simulink model "IEEE30_case"  (R2024b)
settings: Solver=FixedStepAuto  StartTime=0  StopTime=5  FixedStep=1e-7  RelTol=1e-3
values from neighbouring files (symbols this model uses):
  GFL_DFIG_7_C_bus = 0.08    [IEEE30_case_parameters.m]
  GFL_DFIG_7_D_mutual = 2.500000e+3    (= 2500)    [IEEE30_case_parameters.m]
  GFL_DFIG_7_f0 = 60    [IEEE30_case_parameters.m]
  GFL_DFIG_7_gPLLi = 3200    [IEEE30_case_parameters.m]
  GFL_DFIG_7_gPLLp = 650    [IEEE30_case_parameters.m]
  GFL_DFIG_7_H_WT = 0.4    [IEEE30_case_parameters.m]
  GFL_DFIG_7_Hg = 0.8    [IEEE30_case_parameters.m]
  GFL_DFIG_7_Igq_ref = 0    [IEEE30_case_parameters.m]
  GFL_DFIG_7_Ird_ref = 704.45696    [IEEE30_case_parameters.m]
  GFL_DFIG_7_KI_V = -300000    [IEEE30_case_parameters.m]
  GFL_DFIG_7_KP_V = -1000    [IEEE30_case_parameters.m]
  GFL_DFIG_7_Ksh = 1.254300e+4    (= 12543)    [IEEE30_case_parameters.m]
  GFL_DFIG_7_Lg = 0.000483    [IEEE30_case_parameters.m]
  GFL_DFIG_7_Lm_pu = 4    [IEEE30_case_parameters.m]
  GFL_DFIG_7_N = 100    [IEEE30_case_parameters.m]
  GFL_DFIG_7_p = 2    [IEEE30_case_parameters.m]
  GFL_DFIG_7_Pitch = 0    [IEEE30_case_parameters.m]
  GFL_DFIG_7_R = 44    [IEEE30_case_parameters.m]
  GFL_DFIG_7_Rg = 2.000000e-5    (= 2e-05)    [IEEE30_case_parameters.m]
  GFL_DFIG_7_rho = 1.225    [IEEE30_case_parameters.m]
  GFL_DFIG_7_rPLLi = 4500    [IEEE30_case_parameters.m]
  GFL_DFIG_7_rPLLp = 620    [IEEE30_case_parameters.m]
  GFL_DFIG_7_Rs_pu = 0.011    [IEEE30_case_parameters.m]
  GFL_DFIG_7_Sbase = 2.000000e+6    (= 2000000)    [IEEE30_case_parameters.m]
  GFL_DFIG_7_ugq_ref = 0    [IEEE30_case_parameters.m]
  GFL_DFIG_7_usd_ref = 0    [IEEE30_case_parameters.m]
  GFL_DFIG_7_Vbase = 690    [IEEE30_case_parameters.m]
  GFL_DFIG_7_Vdc_ref = 1200    [IEEE30_case_parameters.m]
  GFL_DFIG_7_wind = 12    [IEEE30_case_parameters.m]
  GFL_DFIG_7_wm_ref = 518.184209    [IEEE30_case_parameters.m]
  SG_D_13_D = 0.01056    [IEEE30_case_parameters.m]
  SG_D_13_EnableSaturation = 0    [IEEE30_case_parameters.m]
  SG_D_13_f0 = 60    [IEEE30_case_parameters.m]
  SG_D_13_H = 7.5    [IEEE30_case_parameters.m]
  SG_D_13_K_A = 20    [IEEE30_case_parameters.m]
  SG_D_13_K_E = 1.000000e+1    (= 10)    [IEEE30_case_parameters.m]
  SG_D_13_K_F = 2.363    [IEEE30_case_parameters.m]
  SG_D_13_K_s = 0.5    [IEEE30_case_parameters.m]
  SG_D_13_R_a = 0.001088    [IEEE30_case_parameters.m]
  SG_D_13_S_A = 1    [IEEE30_case_parameters.m]
  SG_D_13_S_B = 0.103    [IEEE30_case_parameters.m]
  SG_D_13_S_N = 10.659857    [IEEE30_case_parameters.m]
  SG_D_13_SpeedPara = 200    [IEEE30_case_parameters.m]
  SG_D_13_T_0 = 0.370163    [IEEE30_case_parameters.m]
  SG_D_13_T_1 = 0.3    [IEEE30_case_parameters.m]
  SG_D_13_T_2 = 0.05    [IEEE30_case_parameters.m]
  SG_D_13_T_3 = 0.02    [IEEE30_case_parameters.m]
  SG_D_13_T_4 = 0.005    [IEEE30_case_parameters.m]
  SG_D_13_T_A = 0.02    [IEEE30_case_parameters.m]
  SG_D_13_T_dd = 8.000000e+0    (= 8)    [IEEE30_case_parameters.m]
  SG_D_13_T_ddd = 0.04    [IEEE30_case_parameters.m]
  SG_D_13_T_E = 0.314    [IEEE30_case_parameters.m]
  SG_D_13_T_F = 0.35    [IEEE30_case_parameters.m]
  SG_D_13_T_qd = 0.8    [IEEE30_case_parameters.m]
  SG_D_13_T_qdd = 0.02    [IEEE30_case_parameters.m]
  SG_D_13_T_speed = 0.1    [IEEE30_case_parameters.m]
  SG_D_13_T_w = 0.5    [IEEE30_case_parameters.m]
  SG_D_13_V_ref = 1.696619    [IEEE30_case_parameters.m]
  SG_D_13_w_ref = 376.991118    [IEEE30_case_parameters.m]
  SG_D_13_x_d = 1.9    [IEEE30_case_parameters.m]
  SG_D_13_x_dd = 0.302    [IEEE30_case_parameters.m]
  SG_D_13_x_ddd = 0.204    [IEEE30_case_parameters.m]
  SG_D_13_x_l = 0.05    [IEEE30_case_parameters.m]
  SG_D_13_x_q = 1.3    [IEEE30_case_parameters.m]
  SG_D_13_x_qd = 0.5    [IEEE30_case_parameters.m]
  SG_D_13_x_qdd = 0.3    [IEEE30_case_parameters.m]
  SG_D_1_D = 0.01056    [IEEE30_case_parameters.m]
  SG_D_1_EnableSaturation = 0    [IEEE30_case_parameters.m]
  SG_D_1_f0 = 60    [IEEE30_case_parameters.m]
  SG_D_1_H = 7.5    [IEEE30_case_parameters.m]
  SG_D_1_K_A = 20    [IEEE30_case_parameters.m]
  SG_D_1_K_E = 1.000000e+1    (= 10)    [IEEE30_case_parameters.m]
  SG_D_1_K_F = 2.363    [IEEE30_case_parameters.m]
  SG_D_1_K_s = 0.5    [IEEE30_case_parameters.m]
  SG_D_1_R_a = 0.001088    [IEEE30_case_parameters.m]
  SG_D_1_S_A = 1    [IEEE30_case_parameters.m]
  SG_D_1_S_B = 0.103    [IEEE30_case_parameters.m]
  SG_D_1_S_N = 10.659857    [IEEE30_case_parameters.m]
  SG_D_1_SpeedPara = 200    [IEEE30_case_parameters.m]
  SG_D_1_T_0 = 0.259812    [IEEE30_case_parameters.m]
  SG_D_1_T_1 = 0.3    [IEEE30_case_parameters.m]
  SG_D_1_T_2 = 0.05    [IEEE30_case_parameters.m]
  SG_D_1_T_3 = 0.02    [IEEE30_case_parameters.m]
  SG_D_1_T_4 = 0.005    [IEEE30_case_parameters.m]
  SG_D_1_T_A = 0.02    [IEEE30_case_parameters.m]
  SG_D_1_T_dd = 8.000000e+0    (= 8)    [IEEE30_case_parameters.m]
  SG_D_1_T_ddd = 0.04    [IEEE30_case_parameters.m]
  SG_D_1_T_E = 0.314    [IEEE30_case_parameters.m]
  SG_D_1_T_F = 0.35    [IEEE30_case_parameters.m]
  SG_D_1_T_qd = 0.8    [IEEE30_case_parameters.m]
  SG_D_1_T_qdd = 0.02    [IEEE30_case_parameters.m]
  SG_D_1_T_speed = 0.1    [IEEE30_case_parameters.m]
  SG_D_1_T_w = 0.5    [IEEE30_case_parameters.m]
  SG_D_1_V_ref = 1.544107    [IEEE30_case_parameters.m]
  SG_D_1_w_ref = 376.991118    [IEEE30_case_parameters.m]
  SG_D_1_x_d = 1.9    [IEEE30_case_parameters.m]
  SG_D_1_x_dd = 0.302    [IEEE30_case_parameters.m]
  SG_D_1_x_ddd = 0.204    [IEEE30_case_parameters.m]
  SG_D_1_x_l = 0.05    [IEEE30_case_parameters.m]
  SG_D_1_x_q = 1.3    [IEEE30_case_parameters.m]
  SG_D_1_x_qd = 0.5    [IEEE30_case_parameters.m]
  SG_D_1_x_qdd = 0.3    [IEEE30_case_parameters.m]
  SG_D_22_D = 0.01056    [IEEE30_case_parameters.m]
  SG_D_22_EnableSaturation = 0    [IEEE30_case_parameters.m]
  SG_D_22_f0 = 60    [IEEE30_case_parameters.m]
  SG_D_22_H = 7.5    [IEEE30_case_parameters.m]
  SG_D_22_K_A = 20    [IEEE30_case_parameters.m]
  SG_D_22_K_E = 1.000000e+1    (= 10)    [IEEE30_case_parameters.m]
  SG_D_22_K_F = 2.363    [IEEE30_case_parameters.m]
  SG_D_22_K_s = 0.5    [IEEE30_case_parameters.m]
  SG_D_22_R_a = 0.001088    [IEEE30_case_parameters.m]
  SG_D_22_S_A = 1    [IEEE30_case_parameters.m]
  SG_D_22_S_B = 0.103    [IEEE30_case_parameters.m]
  SG_D_22_S_N = 10.659857    [IEEE30_case_parameters.m]
  SG_D_22_SpeedPara = 200    [IEEE30_case_parameters.m]
  SG_D_22_T_0 = 0.216121    [IEEE30_case_parameters.m]
  SG_D_22_T_1 = 0.3    [IEEE30_case_parameters.m]
  SG_D_22_T_2 = 0.05    [IEEE30_case_parameters.m]
  SG_D_22_T_3 = 0.02    [IEEE30_case_parameters.m]
  SG_D_22_T_4 = 0.005    [IEEE30_case_parameters.m]
  ... (+126 more)
(part 4 of 27)

== system IEEE30_case/SG_D_22 ==
  v_d_SG_D_22 : Inport
  v_q_SG_D_22 : Inport  Port=2
  E_fd_SG_D_22 : Integrator  InitialCondition=1.7973763049191707
  Px_1_SG_D_22 : Integrator  InitialCondition=0.0
  Px_2_SG_D_22 : Integrator  InitialCondition=0.0
  Px_3_SG_D_22 : Integrator  InitialCondition=9.720418694266681e-32
  R_f_SG_D_22 : Integrator  InitialCondition=12.134857738640001
  T_e_SG_D_22_block : Subsystem
  T_m_SG_D_22 : Integrator  InitialCondition=0.21612107186011983
  V_f_SG_D_22 : Integrator  InitialCondition=17.973763049191707
  d_E_fd_SG_D_22_block : Subsystem
  d_Px_1_SG_D_22_block : Subsystem
  d_Px_2_SG_D_22_block : Subsystem
  d_Px_3_SG_D_22_block : Subsystem
  d_R_f_SG_D_22_block : Subsystem
  d_T_m_SG_D_22_block : Subsystem
  d_V_f_SG_D_22_block : Subsystem
  d_psi_1d_SG_D_22_block : Subsystem
  d_psi_d_SG_D_22_block : Subsystem
  d_psi_fd_SG_D_22_block : Subsystem
  d_psi_gq_SG_D_22_block : Subsystem
  d_psi_kq_SG_D_22_block : Subsystem
  d_psi_q_SG_D_22_block : Subsystem
  d_theta_SG_D_22_block : Subsystem
  d_w_SG_D_22_block : Subsystem
  i_d_SG_D_22_block : Subsystem
  i_q_SG_D_22_block : Subsystem
  psi_1d_SG_D_22 : Integrator  InitialCondition=1.00488248469618
  psi_d_SG_D_22 : Integrator  InitialCondition=0.9834637327982612
  psi_fd_SG_D_22 : Integrator  InitialCondition=1.11283299426169
  psi_gq_SG_D_22 : Integrator  InitialCondition=0.11224508298484515
  psi_kq_SG_D_22 : Integrator  InitialCondition=-0.17538294216382055
  psi_q_SG_D_22 : Integrator  InitialCondition=-0.18239825985037336
  theta_SG_D_22 : Integrator  InitialCondition=0.1237367846423987
  theta_SG_D_22_out_block : Subsystem
  w_SG_D_22 : Integrator  InitialCondition=376.99111843077515
  w_SG_D_22_out_block : Subsystem
  i_d_SG_D_22 : Outport
  i_q_SG_D_22 : Outport  Port=2
  T_e_SG_D_22 : Outport  Port=3
  w_SG_D_22_out : Outport  Port=4
  theta_SG_D_22_out : Outport  Port=5
  wires:
  d_T_m_SG_D_22_block/1(Blockout_d_T_m_SG_D_22_e6732) -> T_m_SG_D_22/1
  psi_kq_SG_D_22/1 -> d_psi_gq_SG_D_22_block/3(State_psi_kq_SG_D_22_f3021), d_psi_q_SG_D_22_block/2(State_psi_kq_SG_D_22_098fe), d_psi_gq_SG_D_22_block/5(State_psi_kq_SG_D_22_d52e6), d_psi_gq_SG_D_22_block/8(State_psi_kq_SG_D_22_c01c1), d_psi_kq_SG_D_22_block/2(State_psi_kq_SG_D_22_eb2c5), i_d_SG_D_22_block/2(State_psi_kq_SG_D_22_d07e7), d_V_f_SG_D_22_block/10(State_psi_kq_SG_D_22_352c2), i_q_SG_D_22_block/2(State_psi_kq_SG_D_22_c8bb0), d_w_SG_D_22_block/5(State_psi_kq_SG_D_22_23ee7), d_psi_kq_SG_D_22_block/4(State_psi_kq_SG_D_22_49ea5), T_e_SG_D_22_block/3(State_psi_kq_SG_D_22_80cd8)
  w_SG_D_22/1 -> d_psi_d_SG_D_22_block/9(State_w_SG_D_22_ad5b4), d_psi_q_SG_D_22_block/9(State_w_SG_D_22_27ecd), d_w_SG_D_22_block/1(State_w_SG_D_22_fa999), d_V_f_SG_D_22_block/13(State_w_SG_D_22_31356), d_V_f_SG_D_22_block/8(State_w_SG_D_22_d59fe), d_theta_SG_D_22_block/1(State_w_SG_D_22_7f5ca), d_T_m_SG_D_22_block/1(State_w_SG_D_22_92dc5), d_Px_1_SG_D_22_block/2(State_w_SG_D_22_b06b5), d_Px_2_SG_D_22_block/4(State_w_SG_D_22_79a8a), d_Px_3_SG_D_22_block/6(State_w_SG_D_22_b3bb6), w_SG_D_22_out_block/1(State_w_SG_D_22_6ca8a)
  d_Px_1_SG_D_22_block/1(Blockout_d_Px_1_SG_D_22_5a954) -> Px_1_SG_D_22/1
  i_q_SG_D_22_block/1(Blockout_i_q_SG_D_22_b8c62) -> i_q_SG_D_22/1
  T_e_SG_D_22_block/1(Blockout_T_e_SG_D_22_9d77c) -> T_e_SG_D_22/1
  psi_gq_SG_D_22/1 -> d_psi_q_SG_D_22_block/1(State_psi_gq_SG_D_22_8eb30), d_psi_gq_SG_D_22_block/1(State_psi_gq_SG_D_22_18129), d_psi_gq_SG_D_22_block/2(State_psi_gq_SG_D_22_c69e2), d_psi_gq_SG_D_22_block/4(State_psi_gq_SG_D_22_61da9), d_psi_kq_SG_D_22_block/1(State_psi_gq_SG_D_22_5f63f), i_d_SG_D_22_block/1(State_psi_gq_SG_D_22_058cc), d_V_f_SG_D_22_block/9(State_psi_gq_SG_D_22_abe45), d_w_SG_D_22_block/4(State_psi_gq_SG_D_22_bb4d3), i_q_SG_D_22_block/1(State_psi_gq_SG_D_22_6529e), d_psi_kq_SG_D_22_block/3(State_psi_gq_SG_D_22_c1d1e), d_psi_gq_SG_D_22_block/7(State_psi_gq_SG_D_22_1b6c4), T_e_SG_D_22_block/2(State_psi_gq_SG_D_22_ecb3d)
  v_q_SG_D_22/1 -> d_psi_d_SG_D_22_block/6(Input_v_q_SG_D_22_3bdb8), d_psi_q_SG_D_22_block/6(Input_v_q_SG_D_22_03d27)
  d_theta_SG_D_22_block/1(Blockout_d_theta_SG_D_22_65d2b) -> theta_SG_D_22/1
  d_Px_3_SG_D_22_block/1(Blockout_d_Px_3_SG_D_22_a3854) -> Px_3_SG_D_22/1
  theta_SG_D_22_out_block/1(Blockout_theta_SG_D_22_out_cf0c5) -> theta_SG_D_22_out/1
  d_Px_2_SG_D_22_block/1(Blockout_d_Px_2_SG_D_22_87151) -> Px_2_SG_D_22/1
  w_SG_D_22_out_block/1(Blockout_w_SG_D_22_out_8ba47) -> w_SG_D_22_out/1
  psi_1d_SG_D_22/1 -> d_psi_fd_SG_D_22_block/3(State_psi_1d_SG_D_22_be8ba), d_psi_fd_SG_D_22_block/8(State_psi_1d_SG_D_22_ea7d2), d_psi_d_SG_D_22_block/1(State_psi_1d_SG_D_22_f0d35), d_psi_1d_SG_D_22_block/1(State_psi_1d_SG_D_22_172da), d_V_f_SG_D_22_block/4(State_psi_1d_SG_D_22_11dba), d_psi_1d_SG_D_22_block/3(State_psi_1d_SG_D_22_e0ab6), d_w_SG_D_22_block/8(State_psi_1d_SG_D_22_62d4d), i_d_SG_D_22_block/5(State_psi_1d_SG_D_22_424d2), d_psi_fd_SG_D_22_block/5(State_psi_1d_SG_D_22_63a8d), i_q_SG_D_22_block/5(State_psi_1d_SG_D_22_666cb), T_e_SG_D_22_block/6(State_psi_1d_SG_D_22_9ed94)
  Px_3_SG_D_22/1 -> d_V_f_SG_D_22_block/3(State_Px_3_SG_D_22_7a9b4), d_Px_3_SG_D_22_block/1(State_Px_3_SG_D_22_2d550)
  theta_SG_D_22/1 -> d_psi_d_SG_D_22_block/5(State_theta_SG_D_22_96219), d_psi_d_SG_D_22_block/7(State_theta_SG_D_22_18f7d), d_psi_q_SG_D_22_block/5(State_theta_SG_D_22_55bda), i_d_SG_D_22_block/4(State_theta_SG_D_22_792f8), i_d_SG_D_22_block/8(State_theta_SG_D_22_e389e), i_q_SG_D_22_block/4(State_theta_SG_D_22_35a4e), i_q_SG_D_22_block/8(State_theta_SG_D_22_5c4fb), theta_SG_D_22_out_block/1(State_theta_SG_D_22_89d34), d_psi_q_SG_D_22_block/7(State_theta_SG_D_22_3fd59)
  Px_2_SG_D_22/1 -> d_Px_3_SG_D_22_block/2(State_Px_2_SG_D_22_afba3), d_Px_3_SG_D_22_block/3(State_Px_2_SG_D_22_1a197), d_Px_2_SG_D_22_block/1(State_Px_2_SG_D_22_a7e01)
  d_psi_kq_SG_D_22_block/1(Blockout_d_psi_kq_SG_D_22_a4b99) -> psi_kq_SG_D_22/1
  psi_d_SG_D_22/1 -> d_psi_fd_SG_D_22_block/9(State_psi_d_SG_D_22_f7c75), d_psi_fd_SG_D_22_block/6(State_psi_d_SG_D_22_1ab68), d_psi_d_SG_D_22_block/2(State_psi_d_SG_D_22_c5170), d_psi_q_SG_D_22_block/8(State_psi_d_SG_D_22_a1733), d_psi_1d_SG_D_22_block/4(State_psi_d_SG_D_22_a4972), d_w_SG_D_22_block/3(State_psi_d_SG_D_22_73560), d_V_f_SG_D_22_block/5(State_psi_d_SG_D_22_b21fa), d_w_SG_D_22_block/9(State_psi_d_SG_D_22_0b647), i_q_SG_D_22_block/6(State_psi_d_SG_D_22_f015b), i_d_SG_D_22_block/6(State_psi_d_SG_D_22_8fd04), T_e_SG_D_22_block/1(State_psi_d_SG_D_22_b0899), T_e_SG_D_22_block/7(State_psi_d_SG_D_22_2f3ed), d_V_f_SG_D_22_block/12(State_psi_d_SG_D_22_8b3f8)
  T_m_SG_D_22/1 -> d_T_m_SG_D_22_block/2(State_T_m_SG_D_22_f2698), d_w_SG_D_22_block/2(State_T_m_SG_D_22_7e244)
  v_d_SG_D_22/1 -> d_psi_d_SG_D_22_block/4(Input_v_d_SG_D_22_73bdd), d_psi_q_SG_D_22_block/4(Input_v_d_SG_D_22_2b34c)
  i_d_SG_D_22_block/1(Blockout_i_d_SG_D_22_9977f) -> i_d_SG_D_22/1
  psi_fd_SG_D_22/1 -> d_psi_fd_SG_D_22_block/4(State_psi_fd_SG_D_22_f44ac), d_psi_fd_SG_D_22_block/7(State_psi_fd_SG_D_22_b3331), d_psi_fd_SG_D_22_block/10(State_psi_fd_SG_D_22_ee685), d_psi_fd_SG_D_22_block/2(State_psi_fd_SG_D_22_5b8ee), d_psi_d_SG_D_22_block/3(State_psi_fd_SG_D_22_05db2), d_psi_1d_SG_D_22_block/2(State_psi_fd_SG_D_22_c2d5a), d_V_f_SG_D_22_block/6(State_psi_fd_SG_D_22_e3f07), i_d_SG_D_22_block/7(State_psi_fd_SG_D_22_0bdd4), d_w_SG_D_22_block/10(State_psi_fd_SG_D_22_b8daa), d_psi_1d_SG_D_22_block/5(State_psi_fd_SG_D_22_3322a), i_q_SG_D_22_block/7(State_psi_fd_SG_D_22_6d852), T_e_SG_D_22_block/8(State_psi_fd_SG_D_22_d61c9)
  psi_q_SG_D_22/1 -> d_psi_d_SG_D_22_block/8(State_psi_q_SG_D_22_e1063), d_psi_q_SG_D_22_block/3(State_psi_q_SG_D_22_dc44e), d_psi_gq_SG_D_22_block/6(State_psi_q_SG_D_22_52758), d_psi_gq_SG_D_22_block/9(State_psi_q_SG_D_22_91585), d_psi_kq_SG_D_22_block/5(State_psi_q_SG_D_22_89f21), d_w_SG_D_22_block/6(State_psi_q_SG_D_22_4ef4a), d_V_f_SG_D_22_block/7(State_psi_q_SG_D_22_f5df1), d_V_f_SG_D_22_block/11(State_psi_q_SG_D_22_c4168), d_w_SG_D_22_block/7(State_psi_q_SG_D_22_8c90d), i_d_SG_D_22_block/3(State_psi_q_SG_D_22_9e84b), T_e_SG_D_22_block/5(State_psi_q_SG_D_22_21d92), T_e_SG_D_22_block/4(State_psi_q_SG_D_22_f98a6), i_q_SG_D_22_block/3(State_psi_q_SG_D_22_a1550)
  Px_1_SG_D_22/1 -> d_Px_2_SG_D_22_block/2(State_Px_1_SG_D_22_e638c), d_Px_3_SG_D_22_block/4(State_Px_1_SG_D_22_68613), d_Px_3_SG_D_22_block/5(State_Px_1_SG_D_22_83b83), d_Px_2_SG_D_22_block/3(State_Px_1_SG_D_22_dd336), d_Px_1_SG_D_22_block/1(State_Px_1_SG_D_22_97642)
  d_E_fd_SG_D_22_block/1(Blockout_d_E_fd_SG_D_22_040cd) -> E_fd_SG_D_22/1
  d_V_f_SG_D_22_block/1(Blockout_d_V_f_SG_D_22_187ed) -> V_f_SG_D_22/1
  d_psi_1d_SG_D_22_block/1(Blockout_d_psi_1d_SG_D_22_39dbc) -> psi_1d_SG_D_22/1
  d_R_f_SG_D_22_block/1(Blockout_d_R_f_SG_D_22_62abf) -> R_f_SG_D_22/1
  d_psi_gq_SG_D_22_block/1(Blockout_d_psi_gq_SG_D_22_8bac2) -> psi_gq_SG_D_22/1
  d_psi_d_SG_D_22_block/1(Blockout_d_psi_d_SG_D_22_244d3) -> psi_d_SG_D_22/1
  d_w_SG_D_22_block/1(Blockout_d_w_SG_D_22_fc61f) -> w_SG_D_22/1
  d_psi_q_SG_D_22_block/1(Blockout_d_psi_q_SG_D_22_d620a) -> psi_q_SG_D_22/1
  R_f_SG_D_22/1 -> d_V_f_SG_D_22_block/2(State_R_f_SG_D_22_2faca), d_R_f_SG_D_22_block/2(State_R_f_SG_D_22_53fbc)
  V_f_SG_D_22/1 -> d_V_f_SG_D_22_block/14(State_V_f_SG_D_22_db965), d_E_fd_SG_D_22_block/2(State_V_f_SG_D_22_c66fa)
  E_fd_SG_D_22/1 -> d_V_f_SG_D_22_block/1(State_E_fd_SG_D_22_743c3), d_E_fd_SG_D_22_block/1(State_E_fd_SG_D_22_b7fa0), d_psi_fd_SG_D_22_block/1(State_E_fd_SG_D_22_516e7), d_R_f_SG_D_22_block/1(State_E_fd_SG_D_22_1081a)
  d_psi_fd_SG_D_22_block/1(Blockout_d_psi_fd_SG_D_22_1ac55) -> psi_fd_SG_D_22/1

== system IEEE30_case/SG_D_23 ==
  v_d_SG_D_23 : Inport
  v_q_SG_D_23 : Inport  Port=2
  E_fd_SG_D_23 : Integrator  InitialCondition=1.2033630369488155
  Px_1_SG_D_23 : Integrator  InitialCondition=0.0
  Px_2_SG_D_23 : Integrator  InitialCondition=0.0
  Px_3_SG_D_23 : Integrator  InitialCondition=-1.0345427304101987e-30
  R_f_SG_D_23 : Integrator  InitialCondition=8.124419589457288
  T_e_SG_D_23_block : Subsystem
  T_m_SG_D_23 : Integrator  InitialCondition=0.19204698605794301
  V_f_SG_D_23 : Integrator  InitialCondition=12.033630369488154
  d_E_fd_SG_D_23_block : Subsystem
  d_Px_1_SG_D_23_block : Subsystem
  d_Px_2_SG_D_23_block : Subsystem
  d_Px_3_SG_D_23_block : Subsystem
  d_R_f_SG_D_23_block : Subsystem
  d_T_m_SG_D_23_block : Subsystem
  d_V_f_SG_D_23_block : Subsystem
  d_psi_1d_SG_D_23_block : Subsystem
  d_psi_d_SG_D_23_block : Subsystem
  d_psi_fd_SG_D_23_block : Subsystem
  d_psi_gq_SG_D_23_block : Subsystem
  d_psi_kq_SG_D_23_block : Subsystem
  d_psi_q_SG_D_23_block : Subsystem
  d_theta_SG_D_23_block : Subsystem
  d_w_SG_D_23_block : Subsystem
  i_d_SG_D_23_block : Subsystem
  i_q_SG_D_23_block : Subsystem
  psi_1d_SG_D_23 : Integrator  InitialCondition=0.9815595669546187
  psi_d_SG_D_23 : Integrator  InitialCondition=0.975564878576397
  psi_fd_SG_D_23 : Integrator  InitialCondition=1.0117727963808552
  psi_gq_SG_D_23 : Integrator  InitialCondition=0.13579101365568608
  psi_kq_SG_D_23 : Integrator  InitialCondition=-0.2121734588370095
  psi_q_SG_D_23 : Integrator  InitialCondition=-0.22066039719048988
  theta_SG_D_23 : Integrator  InitialCondition=0.19462050662964567
  theta_SG_D_23_out_block : Subsystem
  w_SG_D_23 : Integrator  InitialCondition=376.99111843077515
  w_SG_D_23_out_block : Subsystem
  i_d_SG_D_23 : Outport
  i_q_SG_D_23 : Outport  Port=2
  T_e_SG_D_23 : Outport  Port=3
  w_SG_D_23_out : Outport  Port=4
  theta_SG_D_23_out : Outport  Port=5
  wires:
  theta_SG_D_23/1 -> d_psi_d_SG_D_23_block/5(State_theta_SG_D_23_2ec18), d_psi_q_SG_D_23_block/7(State_theta_SG_D_23_99733), i_d_SG_D_23_block/4(State_theta_SG_D_23_46601), i_q_SG_D_23_block/4(State_theta_SG_D_23_c31a3), d_psi_q_SG_D_23_block/5(State_theta_SG_D_23_d0e02), d_psi_d_SG_D_23_block/7(State_theta_SG_D_23_794b5), theta_SG_D_23_out_block/1(State_theta_SG_D_23_9d978), i_q_SG_D_23_block/8(State_theta_SG_D_23_c16ba), i_d_SG_D_23_block/8(State_theta_SG_D_23_15384)
  w_SG_D_23/1 -> d_psi_d_SG_D_23_block/9(State_w_SG_D_23_6d242), d_psi_q_SG_D_23_block/9(State_w_SG_D_23_ea7ff), d_w_SG_D_23_block/1(State_w_SG_D_23_a9c86), d_V_f_SG_D_23_block/13(State_w_SG_D_23_96713), d_V_f_SG_D_23_block/8(State_w_SG_D_23_e30d8), d_theta_SG_D_23_block/1(State_w_SG_D_23_9ae8c), d_T_m_SG_D_23_block/1(State_w_SG_D_23_66b81), d_Px_1_SG_D_23_block/2(State_w_SG_D_23_c0c14), d_Px_2_SG_D_23_block/4(State_w_SG_D_23_f4d00), d_Px_3_SG_D_23_block/6(State_w_SG_D_23_9958b), w_SG_D_23_out_block/1(State_w_SG_D_23_a1e59)
  d_T_m_SG_D_23_block/1(Blockout_d_T_m_SG_D_23_c269a) -> T_m_SG_D_23/1
  V_f_SG_D_23/1 -> d_V_f_SG_D_23_block/14(State_V_f_SG_D_23_beee3), d_E_fd_SG_D_23_block/2(State_V_f_SG_D_23_7cc34)
  d_theta_SG_D_23_block/1(Blockout_d_theta_SG_D_23_51717) -> theta_SG_D_23/1
  w_SG_D_23_out_block/1(Blockout_w_SG_D_23_out_6070a) -> w_SG_D_23_out/1
  i_d_SG_D_23_block/1(Blockout_i_d_SG_D_23_e5d44) -> i_d_SG_D_23/1
  d_Px_1_SG_D_23_block/1(Blockout_d_Px_1_SG_D_23_e26cf) -> Px_1_SG_D_23/1
  psi_1d_SG_D_23/1 -> d_psi_fd_SG_D_23_block/5(State_psi_1d_SG_D_23_20435), d_psi_fd_SG_D_23_block/8(State_psi_1d_SG_D_23_3e436), d_psi_fd_SG_D_23_block/3(State_psi_1d_SG_D_23_a98e3), d_psi_d_SG_D_23_block/1(State_psi_1d_SG_D_23_8965f), d_psi_1d_SG_D_23_block/1(State_psi_1d_SG_D_23_f9ad5), d_w_SG_D_23_block/8(State_psi_1d_SG_D_23_250d1), i_d_SG_D_23_block/5(State_psi_1d_SG_D_23_7111a), i_q_SG_D_23_block/5(State_psi_1d_SG_D_23_19122), d_psi_1d_SG_D_23_block/3(State_psi_1d_SG_D_23_5015b), T_e_SG_D_23_block/6(State_psi_1d_SG_D_23_5b6b0), d_V_f_SG_D_23_block/4(State_psi_1d_SG_D_23_57163)
  psi_fd_SG_D_23/1 -> d_psi_fd_SG_D_23_block/2(State_psi_fd_SG_D_23_a87ca), d_psi_fd_SG_D_23_block/4(State_psi_fd_SG_D_23_d0500), d_psi_fd_SG_D_23_block/10(State_psi_fd_SG_D_23_640f3), d_psi_d_SG_D_23_block/3(State_psi_fd_SG_D_23_f3d1f), d_psi_1d_SG_D_23_block/2(State_psi_fd_SG_D_23_0adb9), d_psi_1d_SG_D_23_block/5(State_psi_fd_SG_D_23_ec5fd), d_w_SG_D_23_block/10(State_psi_fd_SG_D_23_fba26), i_d_SG_D_23_block/7(State_psi_fd_SG_D_23_8232a), d_psi_fd_SG_D_23_block/7(State_psi_fd_SG_D_23_a8ac0), i_q_SG_D_23_block/7(State_psi_fd_SG_D_23_b9ece), d_V_f_SG_D_23_block/6(State_psi_fd_SG_D_23_04b50), T_e_SG_D_23_block/8(State_psi_fd_SG_D_23_2df9d)
  theta_SG_D_23_out_block/1(Blockout_theta_SG_D_23_out_f3dde) -> theta_SG_D_23_out/1
  d_Px_2_SG_D_23_block/1(Blockout_d_Px_2_SG_D_23_c0747) -> Px_2_SG_D_23/1
  psi_kq_SG_D_23/1 -> d_psi_q_SG_D_23_block/2(State_psi_kq_SG_D_23_a5d65), d_psi_gq_SG_D_23_block/3(State_psi_kq_SG_D_23_2d830), d_psi_gq_SG_D_23_block/5(State_psi_kq_SG_D_23_b4351), d_psi_kq_SG_D_23_block/4(State_psi_kq_SG_D_23_31b6f), d_V_f_SG_D_23_block/10(State_psi_kq_SG_D_23_407b5), d_w_SG_D_23_block/5(State_psi_kq_SG_D_23_85da1), i_q_SG_D_23_block/2(State_psi_kq_SG_D_23_d1d5c), i_d_SG_D_23_block/2(State_psi_kq_SG_D_23_a0ec4), d_psi_kq_SG_D_23_block/2(State_psi_kq_SG_D_23_3117e), d_psi_gq_SG_D_23_block/8(State_psi_kq_SG_D_23_c86ae), T_e_SG_D_23_block/3(State_psi_kq_SG_D_23_f7b1e)
  d_Px_3_SG_D_23_block/1(Blockout_d_Px_3_SG_D_23_d0055) -> Px_3_SG_D_23/1
  Px_2_SG_D_23/1 -> d_Px_3_SG_D_23_block/2(State_Px_2_SG_D_23_11635), d_Px_2_SG_D_23_block/1(State_Px_2_SG_D_23_3cd8e), d_Px_3_SG_D_23_block/3(State_Px_2_SG_D_23_48e63)
  Px_3_SG_D_23/1 -> d_V_f_SG_D_23_block/3(State_Px_3_SG_D_23_60fc2), d_Px_3_SG_D_23_block/1(State_Px_3_SG_D_23_753eb)
  v_d_SG_D_23/1 -> d_psi_d_SG_D_23_block/4(Input_v_d_SG_D_23_9e347), d_psi_q_SG_D_23_block/4(Input_v_d_SG_D_23_a1330)
  v_q_SG_D_23/1 -> d_psi_q_SG_D_23_block/6(Input_v_q_SG_D_23_6ddda), d_psi_d_SG_D_23_block/6(Input_v_q_SG_D_23_ae17a)
  psi_q_SG_D_23/1 -> d_psi_d_SG_D_23_block/8(State_psi_q_SG_D_23_bc7c3), d_psi_q_SG_D_23_block/3(State_psi_q_SG_D_23_cf2f8), d_psi_gq_SG_D_23_block/6(State_psi_q_SG_D_23_fd8a2), d_psi_gq_SG_D_23_block/9(State_psi_q_SG_D_23_a58a4), d_psi_kq_SG_D_23_block/5(State_psi_q_SG_D_23_a4607), d_w_SG_D_23_block/7(State_psi_q_SG_D_23_f4578), d_V_f_SG_D_23_block/11(State_psi_q_SG_D_23_b30af), d_w_SG_D_23_block/6(State_psi_q_SG_D_23_ea802), i_d_SG_D_23_block/3(State_psi_q_SG_D_23_9f429), i_q_SG_D_23_block/3(State_psi_q_SG_D_23_c45ba), T_e_SG_D_23_block/4(State_psi_q_SG_D_23_c6c28), d_V_f_SG_D_23_block/7(State_psi_q_SG_D_23_26ce3), T_e_SG_D_23_block/5(State_psi_q_SG_D_23_65500)
  Px_1_SG_D_23/1 -> d_Px_1_SG_D_23_block/1(State_Px_1_SG_D_23_2554a), d_Px_2_SG_D_23_block/2(State_Px_1_SG_D_23_71728), d_Px_2_SG_D_23_block/3(State_Px_1_SG_D_23_4e2ca), d_Px_3_SG_D_23_block/4(State_Px_1_SG_D_23_327f4), d_Px_3_SG_D_23_block/5(State_Px_1_SG_D_23_5f089)
  d_E_fd_SG_D_23_block/1(Blockout_d_E_fd_SG_D_23_20bd2) -> E_fd_SG_D_23/1
  psi_gq_SG_D_23/1 -> d_psi_q_SG_D_23_block/1(State_psi_gq_SG_D_23_36696), d_psi_gq_SG_D_23_block/2(State_psi_gq_SG_D_23_52211), d_psi_gq_SG_D_23_block/4(State_psi_gq_SG_D_23_9dcc3), d_psi_kq_SG_D_23_block/1(State_psi_gq_SG_D_23_ea537), d_w_SG_D_23_block/4(State_psi_gq_SG_D_23_30ca6), d_psi_kq_SG_D_23_block/3(State_psi_gq_SG_D_23_bc7a2), i_q_SG_D_23_block/1(State_psi_gq_SG_D_23_3b4c4), d_psi_gq_SG_D_23_block/7(State_psi_gq_SG_D_23_02c8f), T_e_SG_D_23_block/2(State_psi_gq_SG_D_23_12628), i_d_SG_D_23_block/1(State_psi_gq_SG_D_23_8a76e), d_V_f_SG_D_23_block/9(State_psi_gq_SG_D_23_a55d6), d_psi_gq_SG_D_23_block/1(State_psi_gq_SG_D_23_15800)
  d_psi_fd_SG_D_23_block/1(Blockout_d_psi_fd_SG_D_23_cc715) -> psi_fd_SG_D_23/1
  T_m_SG_D_23/1 -> d_T_m_SG_D_23_block/2(State_T_m_SG_D_23_81d1e), d_w_SG_D_23_block/2(State_T_m_SG_D_23_67386)
  psi_d_SG_D_23/1 -> d_psi_fd_SG_D_23_block/9(State_psi_d_SG_D_23_78162), d_psi_fd_SG_D_23_block/6(State_psi_d_SG_D_23_5a21e), d_w_SG_D_23_block/9(State_psi_d_SG_D_23_77cdf), i_d_SG_D_23_block/6(State_psi_d_SG_D_23_079bd), T_e_SG_D_23_block/1(State_psi_d_SG_D_23_826a4), d_V_f_SG_D_23_block/12(State_psi_d_SG_D_23_86aef), d_w_SG_D_23_block/3(State_psi_d_SG_D_23_cd292), T_e_SG_D_23_block/7(State_psi_d_SG_D_23_8cfae), i_q_SG_D_23_block/6(State_psi_d_SG_D_23_577bb), d_psi_1d_SG_D_23_block/4(State_psi_d_SG_D_23_22f26), d_psi_q_SG_D_23_block/8(State_psi_d_SG_D_23_d98d6), d_V_f_SG_D_23_block/5(State_psi_d_SG_D_23_08a33), d_psi_d_SG_D_23_block/2(State_psi_d_SG_D_23_016fe)
  d_psi_d_SG_D_23_block/1(Blockout_d_psi_d_SG_D_23_781f9) -> psi_d_SG_D_23/1
  T_e_SG_D_23_block/1(Blockout_T_e_SG_D_23_908bc) -> T_e_SG_D_23/1
  d_V_f_SG_D_23_block/1(Blockout_d_V_f_SG_D_23_71fb2) -> V_f_SG_D_23/1
  d_psi_gq_SG_D_23_block/1(Blockout_d_psi_gq_SG_D_23_82b8d) -> psi_gq_SG_D_23/1
  d_psi_kq_SG_D_23_block/1(Blockout_d_psi_kq_SG_D_23_e5927) -> psi_kq_SG_D_23/1
  d_R_f_SG_D_23_block/1(Blockout_d_R_f_SG_D_23_d5fff) -> R_f_SG_D_23/1
  d_psi_1d_SG_D_23_block/1(Blockout_d_psi_1d_SG_D_23_c2996) -> psi_1d_SG_D_23/1
  d_w_SG_D_23_block/1(Blockout_d_w_SG_D_23_057d1) -> w_SG_D_23/1
  d_psi_q_SG_D_23_block/1(Blockout_d_psi_q_SG_D_23_cbd1d) -> psi_q_SG_D_23/1
  i_q_SG_D_23_block/1(Blockout_i_q_SG_D_23_6ad1e) -> i_q_SG_D_23/1
  E_fd_SG_D_23/1 -> d_R_f_SG_D_23_block/1(State_E_fd_SG_D_23_12145), d_E_fd_SG_D_23_block/1(State_E_fd_SG_D_23_30bc4), d_V_f_SG_D_23_block/1(State_E_fd_SG_D_23_02bc8), d_psi_fd_SG_D_23_block/1(State_E_fd_SG_D_23_28355)
  R_f_SG_D_23/1 -> d_V_f_SG_D_23_block/2(State_R_f_SG_D_23_b6bd9), d_R_f_SG_D_23_block/2(State_R_f_SG_D_23_3a056)

== system IEEE30_case/SG_D_27 ==
  v_d_SG_D_27 : Inport
  v_q_SG_D_27 : Inport  Port=2
  E_fd_SG_D_27 : Integrator  InitialCondition=1.2977768781444083
  Px_1_SG_D_27 : Integrator  InitialCondition=0.0
  Px_2_SG_D_27 : Integrator  InitialCondition=0.0
  Px_3_SG_D_27 : Integrator  InitialCondition=3.8336666227978046e-30
  R_f_SG_D_27 : Integrator  InitialCondition=8.761847894443536
  T_e_SG_D_27_block : Subsystem
  T_m_SG_D_27 : Integrator  InitialCondition=0.26919087523977936
  V_f_SG_D_27 : Integrator  InitialCondition=12.977768781444082
  d_E_fd_SG_D_27_block : Subsystem
  d_Px_1_SG_D_27_block : Subsystem
  d_Px_2_SG_D_27_block : Subsystem
  d_Px_3_SG_D_27_block : Subsystem
  d_R_f_SG_D_27_block : Subsystem
  d_T_m_SG_D_27_block : Subsystem
  d_V_f_SG_D_27_block : Subsystem
  d_psi_1d_SG_D_27_block : Subsystem
  d_psi_d_SG_D_27_block : Subsystem
  d_psi_fd_SG_D_27_block : Subsystem
  d_psi_gq_SG_D_27_block : Subsystem
  d_psi_kq_SG_D_27_block : Subsystem
  d_psi_q_SG_D_27_block : Subsystem
  d_theta_SG_D_27_block : Subsystem
  d_w_SG_D_27_block : Subsystem
  i_d_SG_D_27_block : Subsystem
  i_q_SG_D_27_block : Subsystem
  psi_1d_SG_D_27 : Integrator  InitialCondition=0.96507130233546
  psi_d_SG_D_27 : Integrator  InitialCondition=0.9560792597460287
  psi_fd_SG_D_27 : Integrator  InitialCondition=1.0103911969861925
  psi_gq_SG_D_27 : Integrator  InitialCondition=0.18098806741466486
  psi_kq_SG_D_27 : Integrator  InitialCondition=-0.28279385533541385
  psi_q_SG_D_27 : Integrator  InitialCondition=-0.29410560954883036
  theta_SG_D_27 : Integrator  InitialCondition=0.28385589805393974
  theta_SG_D_27_out_block : Subsystem
  w_SG_D_27 : Integrator  InitialCondition=376.99111843077515
  w_SG_D_27_out_block : Subsystem
  i_d_SG_D_27 : Outport
  i_q_SG_D_27 : Outport  Port=2
  T_e_SG_D_27 : Outport  Port=3
  w_SG_D_27_out : Outport  Port=4
  theta_SG_D_27_out : Outport  Port=5
  wires:
  i_d_SG_D_27_block/1(Blockout_i_d_SG_D_27_44f73) -> i_d_SG_D_27/1
  d_Px_1_SG_D_27_block/1(Blockout_d_Px_1_SG_D_27_439b8) -> Px_1_SG_D_27/1
  w_SG_D_27/1 -> d_w_SG_D_27_block/1(State_w_SG_D_27_b6b9b), d_V_f_SG_D_27_block/8(State_w_SG_D_27_ac390), d_psi_q_SG_D_27_block/9(State_w_SG_D_27_1f9a9), d_V_f_SG_D_27_block/13(State_w_SG_D_27_f905c), d_psi_d_SG_D_27_block/9(State_w_SG_D_27_e9387), d_theta_SG_D_27_block/1(State_w_SG_D_27_a39e4), d_T_m_SG_D_27_block/1(State_w_SG_D_27_b53f8), d_Px_3_SG_D_27_block/6(State_w_SG_D_27_62987), w_SG_D_27_out_block/1(State_w_SG_D_27_8ae81), d_Px_2_SG_D_27_block/4(State_w_SG_D_27_5c50a), d_Px_1_SG_D_27_block/2(State_w_SG_D_27_cf173)
  d_theta_SG_D_27_block/1(Blockout_d_theta_SG_D_27_c4116) -> theta_SG_D_27/1
  psi_d_SG_D_27/1 -> d_psi_fd_SG_D_27_block/6(State_psi_d_SG_D_27_fdc2b), d_psi_fd_SG_D_27_block/9(State_psi_d_SG_D_27_0dbb0), d_psi_d_SG_D_27_block/2(State_psi_d_SG_D_27_a7f1f), d_psi_q_SG_D_27_block/8(State_psi_d_SG_D_27_cb123), d_psi_1d_SG_D_27_block/4(State_psi_d_SG_D_27_a8139), i_d_SG_D_27_block/6(State_psi_d_SG_D_27_2629b), d_V_f_SG_D_27_block/5(State_psi_d_SG_D_27_7c091), d_w_SG_D_27_block/9(State_psi_d_SG_D_27_61c40), i_q_SG_D_27_block/6(State_psi_d_SG_D_27_bea5b), d_V_f_SG_D_27_block/12(State_psi_d_SG_D_27_c8afe), d_w_SG_D_27_block/3(State_psi_d_SG_D_27_07f9f), T_e_SG_D_27_block/7(State_psi_d_SG_D_27_1e6e0), T_e_SG_D_27_block/1(State_psi_d_SG_D_27_aae51)
  d_Px_2_SG_D_27_block/1(Blockout_d_Px_2_SG_D_27_55afa) -> Px_2_SG_D_27/1
  d_T_m_SG_D_27_block/1(Blockout_d_T_m_SG_D_27_75196) -> T_m_SG_D_27/1
  psi_fd_SG_D_27/1 -> d_psi_fd_SG_D_27_block/2(State_psi_fd_SG_D_27_68608), d_psi_fd_SG_D_27_block/4(State_psi_fd_SG_D_27_f02f4), d_psi_fd_SG_D_27_block/7(State_psi_fd_SG_D_27_a093b), d_psi_fd_SG_D_27_block/10(State_psi_fd_SG_D_27_a19a0), d_psi_d_SG_D_27_block/3(State_psi_fd_SG_D_27_62224), d_psi_1d_SG_D_27_block/5(State_psi_fd_SG_D_27_15400), d_psi_1d_SG_D_27_block/2(State_psi_fd_SG_D_27_72b20), d_V_f_SG_D_27_block/6(State_psi_fd_SG_D_27_27c3c), i_d_SG_D_27_block/7(State_psi_fd_SG_D_27_68d93), i_q_SG_D_27_block/7(State_psi_fd_SG_D_27_8eaba), T_e_SG_D_27_block/8(State_psi_fd_SG_D_27_93998), d_w_SG_D_27_block/10(State_psi_fd_SG_D_27_c8345)
  d_Px_3_SG_D_27_block/1(Blockout_d_Px_3_SG_D_27_484b3) -> Px_3_SG_D_27/1
  T_e_SG_D_27_block/1(Blockout_T_e_SG_D_27_0afee) -> T_e_SG_D_27/1
  w_SG_D_27_out_block/1(Blockout_w_SG_D_27_out_337ec) -> w_SG_D_27_out/1
  psi_q_SG_D_27/1 -> d_psi_d_SG_D_27_block/8(State_psi_q_SG_D_27_a07c2), d_psi_gq_SG_D_27_block/6(State_psi_q_SG_D_27_a0060), d_psi_gq_SG_D_27_block/9(State_psi_q_SG_D_27_f7919), d_psi_kq_SG_D_27_block/5(State_psi_q_SG_D_27_76fbd), d_V_f_SG_D_27_block/11(State_psi_q_SG_D_27_7ebac), d_V_f_SG_D_27_block/7(State_psi_q_SG_D_27_dd61c), i_d_SG_D_27_block/3(State_psi_q_SG_D_27_720da), i_q_SG_D_27_block/3(State_psi_q_SG_D_27_1d36b), d_psi_q_SG_D_27_block/3(State_psi_q_SG_D_27_3920f), T_e_SG_D_27_block/4(State_psi_q_SG_D_27_c3716), T_e_SG_D_27_block/5(State_psi_q_SG_D_27_f2155), d_w_SG_D_27_block/7(State_psi_q_SG_D_27_5c8dd), d_w_SG_D_27_block/6(State_psi_q_SG_D_27_b32ea)
  psi_gq_SG_D_27/1 -> d_psi_q_SG_D_27_block/1(State_psi_gq_SG_D_27_e40b4), d_psi_gq_SG_D_27_block/1(State_psi_gq_SG_D_27_c3af2), d_psi_gq_SG_D_27_block/2(State_psi_gq_SG_D_27_6e8f7), d_psi_kq_SG_D_27_block/3(State_psi_gq_SG_D_27_ed697), d_V_f_SG_D_27_block/9(State_psi_gq_SG_D_27_6c126), i_d_SG_D_27_block/1(State_psi_gq_SG_D_27_d72b2), d_psi_gq_SG_D_27_block/4(State_psi_gq_SG_D_27_3e2b9), d_psi_gq_SG_D_27_block/7(State_psi_gq_SG_D_27_ed82f), i_q_SG_D_27_block/1(State_psi_gq_SG_D_27_0dda8), d_w_SG_D_27_block/4(State_psi_gq_SG_D_27_3064d), d_psi_kq_SG_D_27_block/1(State_psi_gq_SG_D_27_3d919), T_e_SG_D_27_block/2(State_psi_gq_SG_D_27_2222e)
  psi_1d_SG_D_27/1 -> d_psi_fd_SG_D_27_block/3(State_psi_1d_SG_D_27_49a09), d_psi_fd_SG_D_27_block/5(State_psi_1d_SG_D_27_946b5), d_psi_fd_SG_D_27_block/8(State_psi_1d_SG_D_27_1e075), d_psi_d_SG_D_27_block/1(State_psi_1d_SG_D_27_d5c1b), d_psi_1d_SG_D_27_block/3(State_psi_1d_SG_D_27_d0b37), d_w_SG_D_27_block/8(State_psi_1d_SG_D_27_4e688), i_q_SG_D_27_block/5(State_psi_1d_SG_D_27_1a223), i_d_SG_D_27_block/5(State_psi_1d_SG_D_27_ec66c), d_V_f_SG_D_27_block/4(State_psi_1d_SG_D_27_082ae), d_psi_1d_SG_D_27_block/1(State_psi_1d_SG_D_27_efe98), T_e_SG_D_27_block/6(State_psi_1d_SG_D_27_3beb4)
  Px_2_SG_D_27/1 -> d_Px_2_SG_D_27_block/1(State_Px_2_SG_D_27_373db), d_Px_3_SG_D_27_block/2(State_Px_2_SG_D_27_7e14b), d_Px_3_SG_D_27_block/3(State_Px_2_SG_D_27_a8fab)
  E_fd_SG_D_27/1 -> d_V_f_SG_D_27_block/1(State_E_fd_SG_D_27_11911), d_R_f_SG_D_27_block/1(State_E_fd_SG_D_27_e31da), d_E_fd_SG_D_27_block/1(State_E_fd_SG_D_27_823cb), d_psi_fd_SG_D_27_block/1(State_E_fd_SG_D_27_fdb39)
  Px_1_SG_D_27/1 -> d_Px_1_SG_D_27_block/1(State_Px_1_SG_D_27_e0716), d_Px_3_SG_D_27_block/4(State_Px_1_SG_D_27_bbb95), d_Px_2_SG_D_27_block/2(State_Px_1_SG_D_27_13dd5), d_Px_2_SG_D_27_block/3(State_Px_1_SG_D_27_849c9), d_Px_3_SG_D_27_block/5(State_Px_1_SG_D_27_e5cc3)
  psi_kq_SG_D_27/1 -> d_psi_q_SG_D_27_block/2(State_psi_kq_SG_D_27_de047), d_psi_gq_SG_D_27_block/3(State_psi_kq_SG_D_27_7c836), d_psi_gq_SG_D_27_block/5(State_psi_kq_SG_D_27_4dbff), i_d_SG_D_27_block/2(State_psi_kq_SG_D_27_7b606), d_w_SG_D_27_block/5(State_psi_kq_SG_D_27_cb932), i_q_SG_D_27_block/2(State_psi_kq_SG_D_27_df7da), d_psi_kq_SG_D_27_block/4(State_psi_kq_SG_D_27_59b97), d_V_f_SG_D_27_block/10(State_psi_kq_SG_D_27_28d7a), d_psi_gq_SG_D_27_block/8(State_psi_kq_SG_D_27_09d28), T_e_SG_D_27_block/3(State_psi_kq_SG_D_27_9e25d), d_psi_kq_SG_D_27_block/2(State_psi_kq_SG_D_27_bbdd7)
  theta_SG_D_27/1 -> d_psi_d_SG_D_27_block/5(State_theta_SG_D_27_17b48), d_psi_d_SG_D_27_block/7(State_theta_SG_D_27_9f539), d_psi_q_SG_D_27_block/7(State_theta_SG_D_27_d8fdd), i_d_SG_D_27_block/4(State_theta_SG_D_27_3e79c), i_q_SG_D_27_block/8(State_theta_SG_D_27_83f88), i_q_SG_D_27_block/4(State_theta_SG_D_27_54b2e), theta_SG_D_27_out_block/1(State_theta_SG_D_27_c2ad6), d_psi_q_SG_D_27_block/5(State_theta_SG_D_27_7e859), i_d_SG_D_27_block/8(State_theta_SG_D_27_e4dee)
  T_m_SG_D_27/1 -> d_T_m_SG_D_27_block/2(State_T_m_SG_D_27_0f28d), d_w_SG_D_27_block/2(State_T_m_SG_D_27_aac0d)
  Px_3_SG_D_27/1 -> d_V_f_SG_D_27_block/3(State_Px_3_SG_D_27_cca99), d_Px_3_SG_D_27_block/1(State_Px_3_SG_D_27_7eb86)
  d_R_f_SG_D_27_block/1(Blockout_d_R_f_SG_D_27_9dd2c) -> R_f_SG_D_27/1
  v_d_SG_D_27/1 -> d_psi_q_SG_D_27_block/4(Input_v_d_SG_D_27_8244b), d_psi_d_SG_D_27_block/4(Input_v_d_SG_D_27_222f7)
  V_f_SG_D_27/1 -> d_V_f_SG_D_27_block/14(State_V_f_SG_D_27_03782), d_E_fd_SG_D_27_block/2(State_V_f_SG_D_27_0da35)
  v_q_SG_D_27/1 -> d_psi_d_SG_D_27_block/6(Input_v_q_SG_D_27_3207e), d_psi_q_SG_D_27_block/6(Input_v_q_SG_D_27_5a914)
  i_q_SG_D_27_block/1(Blockout_i_q_SG_D_27_b805d) -> i_q_SG_D_27/1
  d_V_f_SG_D_27_block/1(Blockout_d_V_f_SG_D_27_ad652) -> V_f_SG_D_27/1
  d_psi_q_SG_D_27_block/1(Blockout_d_psi_q_SG_D_27_cf824) -> psi_q_SG_D_27/1
  d_w_SG_D_27_block/1(Blockout_d_w_SG_D_27_0fca4) -> w_SG_D_27/1
  d_psi_gq_SG_D_27_block/1(Blockout_d_psi_gq_SG_D_27_e3839) -> psi_gq_SG_D_27/1
  d_psi_kq_SG_D_27_block/1(Blockout_d_psi_kq_SG_D_27_1e68d) -> psi_kq_SG_D_27/1
  d_psi_d_SG_D_27_block/1(Blockout_d_psi_d_SG_D_27_ed15c) -> psi_d_SG_D_27/1
  d_psi_1d_SG_D_27_block/1(Blockout_d_psi_1d_SG_D_27_6915f) -> psi_1d_SG_D_27/1
  theta_SG_D_27_out_block/1(Blockout_theta_SG_D_27_out_fd4a4) -> theta_SG_D_27_out/1
  R_f_SG_D_27/1 -> d_V_f_SG_D_27_block/2(State_R_f_SG_D_27_2a887), d_R_f_SG_D_27_block/2(State_R_f_SG_D_27_31c67)
  d_E_fd_SG_D_27_block/1(Blockout_d_E_fd_SG_D_27_b9ef8) -> E_fd_SG_D_27/1
  d_psi_fd_SG_D_27_block/1(Blockout_d_psi_fd_SG_D_27_836bf) -> psi_fd_SG_D_27/1

== system IEEE30_case/Subsystem1 ==
  uq : Inport
  ud : Inport  Port=2
  id : Inport  Port=3
  iq : Inport  Port=4
  Subsystem : Subsystem
  Subsystem1 : Subsystem
  Out1 : Outport
  Out2 : Outport  Port=2
  wires:
  id/1 -> Subsystem/3(id), Subsystem1/1(id)
  ud/1 -> Subsystem/2(ud), Subsystem1/3(ud)
  iq/1 -> Subsystem/4(iq), Subsystem1/2(iq)
  uq/1 -> Subsystem/1(uq), Subsystem1/4(uq)
  Subsystem1/1(Out1) -> Out2/1
  Subsystem/1(Out1) -> Out1/1

== system IEEE30_case/Subsystem2 ==
  uq : Inport
  ud : Inport  Port=2
  id : Inport  Port=3
  iq : Inport  Port=4
  Subsystem : Subsystem
  Subsystem1 : Subsystem
  Out1 : Outport
  Out2 : Outport  Port=2
  wires:
  id/1 -> Subsystem/3(id), Subsystem1/1(id)
  ud/1 -> Subsystem/2(ud), Subsystem1/3(ud)
  iq/1 -> Subsystem/4(iq), Subsystem1/2(iq)
  uq/1 -> Subsystem/1(uq), Subsystem1/4(uq)
  Subsystem1/1(Out1) -> Out2/1
  Subsystem/1(Out1) -> Out1/1

== system IEEE30_case/Subsystem3 ==
  uq : Inport
  ud : Inport  Port=2
  id : Inport  Port=3
  iq : Inport  Port=4
  Subsystem : Subsystem
  Subsystem1 : Subsystem
  Out1 : Outport
  Out2 : Outport  Port=2
  wires:
  id/1 -> Subsystem/3(id), Subsystem1/1(id)
  ud/1 -> Subsystem/2(ud), Subsystem1/3(ud)
  iq/1 -> Subsystem/4(iq), Subsystem1/2(iq)
  uq/1 -> Subsystem/1(uq), Subsystem1/4(uq)
  Subsystem1/1(Out1) -> Out2/1
  Subsystem/1(Out1) -> Out1/1

== system IEEE30_case/Subsystem4 ==
  uq : Inport
  ud : Inport  Port=2
  id : Inport  Port=3
  iq : Inport  Port=4
  Subsystem : Subsystem
  Subsystem1 : Subsystem
  Out1 : Outport
  Out2 : Outport  Port=2
  wires:
  Subsystem/1(Out1) -> Out1/1
  Subsystem1/1(Out1) -> Out2/1
  uq/1 -> Subsystem1/4(uq), Subsystem/1(uq)
  iq/1 -> Subsystem1/2(iq), Subsystem/4(iq)
  ud/1 -> Subsystem1/3(ud), Subsystem/2(ud)
  id/1 -> Subsystem1/1(id), Subsystem/3(id)

== system IEEE30_case/Subsystem5 ==
  uq : Inport
  ud : Inport  Port=2
  id : Inport  Port=3
  iq : Inport  Port=4
  Subsystem : Subsystem
  Subsystem1 : Subsystem
  Out1 : Outport
  Out2 : Outport  Port=2
  wires:
  id/1 -> Subsystem/3(id), Subsystem1/1(id)
  ud/1 -> Subsystem/2(ud), Subsystem1/3(ud)
  iq/1 -> Subsystem/4(iq), Subsystem1/2(iq)
  uq/1 -> Subsystem/1(uq), Subsystem1/4(uq)
  Subsystem1/1(Out1) -> Out2/1
  Subsystem/1(Out1) -> Out1/1

== system IEEE30_case/Subsystem6 ==
  uq : Inport
  ud : Inport  Port=2
  id : Inport  Port=3
  iq : Inport  Port=4
  Subsystem : Subsystem
  Subsystem1 : Subsystem
  Out1 : Outport
  Out2 : Outport  Port=2
  wires:
  id/1 -> Subsystem/3(id), Subsystem1/1(id)
  ud/1 -> Subsystem/2(ud), Subsystem1/3(ud)
  iq/1 -> Subsystem/4(iq), Subsystem1/2(iq)
  uq/1 -> Subsystem/1(uq), Subsystem1/4(uq)
  Subsystem1/1(Out1) -> Out2/1
  Subsystem/1(Out1) -> Out1/1

== system IEEE30_case/Subsystem7 ==
  uq : Inport
  ud : Inport  Port=2
  id : Inport  Port=3
  iq : Inport  Port=4
  Subsystem : Subsystem
  Subsystem1 : Subsystem
  Out1 : Outport
  Out2 : Outport  Port=2
  wires:
  Subsystem/1(Out1) -> Out1/1
  Subsystem1/1(Out1) -> Out2/1
  uq/1 -> Subsystem1/4(uq), Subsystem/1(uq)
  iq/1 -> Subsystem1/2(iq), Subsystem/4(iq)
  ud/1 -> Subsystem1/3(ud), Subsystem/2(ud)
  id/1 -> Subsystem1/1(id), Subsystem/3(id)

== system IEEE30_case/Subsystem8 ==
  tt : Inport
  ft : Inport  Port=2
  tv : Inport  Port=3
  fv : Inport  Port=4
  Clock : Clock
  Minus : Sum  Inputs=+-
  Minus1 : Sum  Inputs=+-
  Switch : Switch  Criteria=u2 > Threshold  SaturateOnIntegerOverflow=off  InputSameDT=off
  Switch1 : Switch  Criteria=u2 > Threshold  SaturateOnIntegerOverflow=off  InputSameDT=off
  Out1 : Outport
  wires:
  ft/1 -> Minus/2
  Switch/1 -> Switch1/3
  Clock/1 -> Minus1/1, Minus/1
  Minus1/1 -> Switch1/2
  Switch1/1 -> Out1/1
  Minus/1 -> Switch/2
  fv/1 -> Switch1/1, Switch/3
  tt/1 -> Minus1/2
  tv/1 -> Switch/1

== system IEEE30_case/AC_1/d_id_line_10_17_block ==
  note: d_id_line_10_17 in IEEE30_case
      | $376.991118430775\,\mathrm{iq}_{\mathrm{line},10,17}-141.371669411541\,\mathrm{id}_{\mathrm{line},10,17}+4712.38898038469\,\mathrm{vd}_{\mathrm{bus},10}-4712.38898038469\,\mathrm{vd}_{\mathrm{bus},17}$
      | Automatically generated on 2025-11-01 18:41:54 .
  State_id_line_10_17_9d65e : Inport
  State_iq_line_10_17_8c10e : Inport  Port=2
  State_vd_bus_10_ba0ab : Inport  Port=3
  State_vd_bus_17_0c9ca : Inport  Port=4
  Add_2e212 : Sum
  Add_6e79c : Sum
  Constant_-141.371669411541_2c7d3 : Constant  Value=-141.371669411541
  Constant_376.991118430775_8875c : Constant  Value=376.991118430775
  Constant_4712.38898038469_1f47d : Constant  Value=4712.38898038469
  Constant_4712.38898038469_e0e8c : Constant  Value=4712.38898038469
  Product_110c2 : Product
  Product_5b4f7 : Product
  Product_62580 : Product
  Product_a0513 : Product
  Subtract_ca9c4 : Sum  Inputs=+-
  Blockout_d_id_line_10_17_512b4 : Outport
  wires:
  Constant_-141.371669411541_2c7d3/1 -> Product_62580/1
  State_id_line_10_17_9d65e/1 -> Product_62580/2
  Constant_376.991118430775_8875c/1 -> Product_5b4f7/1
  State_iq_line_10_17_8c10e/1 -> Product_5b4f7/2
  Product_62580/1 -> Add_6e79c/1
  Product_5b4f7/1 -> Add_6e79c/2
  State_vd_bus_10_ba0ab/1 -> Product_a0513/2
  Product_a0513/1 -> Add_2e212/2
  Constant_4712.38898038469_1f47d/1 -> Product_a0513/1
  Add_6e79c/1 -> Add_2e212/1
  Product_110c2/1 -> Subtract_ca9c4/2
  Constant_4712.38898038469_e0e8c/1 -> Product_110c2/1
  State_vd_bus_17_0c9ca/1 -> Product_110c2/2
  Add_2e212/1 -> Subtract_ca9c4/1
  Subtract_ca9c4/1 -> Blockout_d_id_line_10_17_512b4/1

== system IEEE30_case/AC_1/d_id_line_10_20_block ==
  note: d_id_line_10_20 in IEEE30_case
      | $376.991118430775\,\mathrm{iq}_{\mathrm{line},10,20}-161.567622184618\,\mathrm{id}_{\mathrm{line},10,20}+1795.19580205131\,\mathrm{vd}_{\mathrm{bus},10}-1795.19580205131\,\mathrm{vd}_{\mathrm{bus},20}$
      | Automatically generated on 2025-11-01 18:41:52 .
  State_id_line_10_20_265b4 : Inport
  State_iq_line_10_20_a2259 : Inport  Port=2
  State_vd_bus_10_a2605 : Inport  Port=3
  State_vd_bus_20_a0401 : Inport  Port=4
  Add_e4c1e : Sum
  Add_fc5aa : Sum
  Constant_-161.567622184618_c89c3 : Constant  Value=-161.567622184618
  Constant_1795.19580205131_12fa4 : Constant  Value=1795.19580205131
  Constant_1795.19580205131_87c29 : Constant  Value=1795.19580205131
  Constant_376.991118430775_e8bf0 : Constant  Value=376.991118430775
  Product_3e701 : Product
  Product_52c8d : Product
  Product_908ff : Product
  Product_cd957 : Product
  Subtract_61c13 : Sum  Inputs=+-
  Blockout_d_id_line_10_20_f93f3 : Outport
  wires:
  Constant_-161.567622184618_c89c3/1 -> Product_3e701/1
  Constant_376.991118430775_e8bf0/1 -> Product_cd957/1
  Product_cd957/1 -> Add_fc5aa/2
  Product_3e701/1 -> Add_fc5aa/1
  State_id_line_10_20_265b4/1 -> Product_3e701/2
  Subtract_61c13/1 -> Blockout_d_id_line_10_20_f93f3/1
  State_iq_line_10_20_a2259/1 -> Product_cd957/2
  Product_908ff/1 -> Add_e4c1e/2
  Constant_1795.19580205131_12fa4/1 -> Product_908ff/1
  State_vd_bus_10_a2605/1 -> Product_908ff/2
  Add_fc5aa/1 -> Add_e4c1e/1
  Constant_1795.19580205131_87c29/1 -> Product_52c8d/1
  State_vd_bus_20_a0401/1 -> Product_52c8d/2
  Add_e4c1e/1 -> Subtract_61c13/1
  Product_52c8d/1 -> Subtract_61c13/2

== system IEEE30_case/AC_1/d_id_line_10_21_block ==
  note: d_id_line_10_21 in IEEE30_case
      | $376.991118430775\,\mathrm{iq}_{\mathrm{line},10,21}-161.567622184618\,\mathrm{id}_{\mathrm{line},10,21}+5385.58740615393\,\mathrm{vd}_{\mathrm{bus},10}-5385.58740615393\,\mathrm{vd}_{\mathrm{bus},21}$
      | Automatically generated on 2025-11-01 18:41:56 .
  State_id_line_10_21_d3f7b : Inport
  State_iq_line_10_21_aacb6 : Inport  Port=2
  State_vd_bus_10_3ade5 : Inport  Port=3
  State_vd_bus_21_53c66 : Inport  Port=4
  Add_1d696 : Sum
  Add_5964b : Sum
  Constant_-161.567622184618_561d8 : Constant  Value=-161.567622184618
  Constant_376.991118430775_ddcac : Constant  Value=376.991118430775
  Constant_5385.58740615393_1f2b5 : Constant  Value=5385.58740615393
  Constant_5385.58740615393_b14c4 : Constant  Value=5385.58740615393
  Product_02815 : Product
  Product_0e691 : Product
  Product_3eb27 : Product
  Product_a7c80 : Product
  Subtract_6440e : Sum  Inputs=+-
  Blockout_d_id_line_10_21_8be6c : Outport
  wires:
  Constant_-161.567622184618_561d8/1 -> Product_02815/1
  Constant_5385.58740615393_b14c4/1 -> Product_a7c80/1
  Subtract_6440e/1 -> Blockout_d_id_line_10_21_8be6c/1
  State_id_line_10_21_d3f7b/1 -> Product_02815/2
  Constant_376.991118430775_ddcac/1 -> Product_0e691/1
  Product_0e691/1 -> Add_5964b/2
  State_iq_line_10_21_aacb6/1 -> Product_0e691/2
  Product_02815/1 -> Add_5964b/1
  State_vd_bus_10_3ade5/1 -> Product_a7c80/2
  Add_5964b/1 -> Add_1d696/1
  Product_a7c80/1 -> Add_1d696/2
  Product_3eb27/1 -> Subtract_6440e/2
  Constant_5385.58740615393_1f2b5/1 -> Product_3eb27/1
  State_vd_bus_21_53c66/1 -> Product_3eb27/2
  Add_1d696/1 -> Subtract_6440e/1

== system IEEE30_case/AC_1/d_id_line_10_22_block ==
  note: d_id_line_10_22 in IEEE30_case
      | $376.991118430775\,\mathrm{iq}_{\mathrm{line},10,22}-175.929188601028\,\mathrm{id}_{\mathrm{line},10,22}+2513.27412287183\,\mathrm{vd}_{\mathrm{bus},10}-2513.27412287183\,\mathrm{vd}_{\mathrm{bus},22}$
      | Automatically generated on 2025-11-01 18:41:59 .
  State_id_line_10_22_89fbc : Inport
  State_iq_line_10_22_73dd3 : Inport  Port=2
  State_vd_bus_10_b72dc : Inport  Port=3
  State_vd_bus_22_ced80 : Inport  Port=4
  Add_20305 : Sum
  Add_68c07 : Sum
  Constant_-175.929188601028_b122d : Constant  Value=-175.929188601028
  Constant_2513.27412287183_382a4 : Constant  Value=2513.27412287183
  Constant_2513.27412287183_5be00 : Constant  Value=2513.27412287183
  Constant_376.991118430775_31bad : Constant  Value=376.991118430775
  Product_4a5e0 : Product
  Product_65ad9 : Product
  Product_9b90c : Product
  Product_df0de : Product
  Subtract_ed368 : Sum  Inputs=+-
  Blockout_d_id_line_10_22_d0b41 : Outport
  wires:
  State_vd_bus_22_ced80/1 -> Product_4a5e0/2
  Constant_-175.929188601028_b122d/1 -> Product_65ad9/1
  State_id_line_10_22_89fbc/1 -> Product_65ad9/2
  Constant_376.991118430775_31bad/1 -> Product_9b90c/1
  Product_9b90c/1 -> Add_68c07/2
  Product_df0de/1 -> Add_20305/2
  Constant_2513.27412287183_382a4/1 -> Product_df0de/1
  Subtract_ed368/1 -> Blockout_d_id_line_10_22_d0b41/1
  State_iq_line_10_22_73dd3/1 -> Product_9b90c/2
  Product_65ad9/1 -> Add_68c07/1
  State_vd_bus_10_b72dc/1 -> Product_df0de/2
  Add_68c07/1 -> Add_20305/1
  Product_4a5e0/1 -> Subtract_ed368/2
  Constant_2513.27412287183_5be00/1 -> Product_4a5e0/1
  Add_20305/1 -> Subtract_ed368/1

== system IEEE30_case/AC_1/d_id_line_12_13_block ==
  note: d_id_line_12_13 in IEEE30_case
      | $376.991118430775\,\mathrm{iq}_{\mathrm{line},12,13}+2692.79370307697\,\mathrm{vd}_{\mathrm{bus},12}-2692.79370307697\,\mathrm{vd}_{\mathrm{bus},13}$
      | Automatically generated on 2025-11-01 18:41:31 .
  State_iq_line_12_13_e9023 : Inport
  State_vd_bus_12_4b72e : Inport  Port=2
  State_vd_bus_13_6c93a : Inport  Port=3
  Add_438b1 : Sum
  Constant_2692.79370307697_6588e : Constant  Value=2692.79370307697
  Constant_2692.79370307697_d0b44 : Constant  Value=2692.79370307697
  Constant_376.991118430775_116b5 : Constant  Value=376.991118430775
  Product_2af9b : Product
  Product_89211 : Product
  Product_8dc1b : Product
  Subtract_ba098 : Sum  Inputs=+-
  Blockout_d_id_line_12_13_70d92 : Outport
  wires:
  Constant_376.991118430775_116b5/1 -> Product_8dc1b/1
  Constant_2692.79370307697_6588e/1 -> Product_2af9b/1
  Product_2af9b/1 -> Add_438b1/2
  State_iq_line_12_13_e9023/1 -> Product_8dc1b/2
  State_vd_bus_12_4b72e/1 -> Product_2af9b/2
  Product_8dc1b/1 -> Add_438b1/1
  Constant_2692.79370307697_d0b44/1 -> Product_89211/1
  State_vd_bus_13_6c93a/1 -> Product_89211/2
  Add_438b1/1 -> Subtract_ba098/1
  Product_89211/1 -> Subtract_ba098/2
  Subtract_ba098/1 -> Blockout_d_id_line_12_13_70d92/1

== system IEEE30_case/AC_1/d_id_line_12_14_block ==
  note: d_id_line_12_14 in IEEE30_case
      | $376.991118430775\,\mathrm{iq}_{\mathrm{line},12,14}-173.995900814204\,\mathrm{id}_{\mathrm{line},12,14}+1449.96584011837\,\mathrm{vd}_{\mathrm{bus},12}-1449.96584011837\,\mathrm{vd}_{\mathrm{bus},14}$
      | Automatically generated on 2025-11-01 18:41:33 .
  State_id_line_12_14_67792 : Inport
  State_iq_line_12_14_78bfe : Inport  Port=2
  State_vd_bus_12_691f6 : Inport  Port=3
  State_vd_bus_14_de14e : Inport  Port=4
  Add_25c3a : Sum
  Add_43ae3 : Sum
  Constant_-173.995900814204_48b5e : Constant  Value=-173.995900814204
  Constant_1449.96584011837_14eb9 : Constant  Value=1449.96584011837
  Constant_1449.96584011837_c1ff0 : Constant  Value=1449.96584011837
  Constant_376.991118430775_02c44 : Constant  Value=376.991118430775
  Product_461d6 : Product
  Product_896d7 : Product
  Product_9d282 : Product
  Product_f6103 : Product
  Subtract_29005 : Sum  Inputs=+-
  Blockout_d_id_line_12_14_0b4f3 : Outport
  wires:
  Constant_-173.995900814204_48b5e/1 -> Product_f6103/1
  Product_f6103/1 -> Add_25c3a/1
  State_id_line_12_14_67792/1 -> Product_f6103/2
  Constant_376.991118430775_02c44/1 -> Product_896d7/1
  Product_896d7/1 -> Add_25c3a/2
  State_iq_line_12_14_78bfe/1 -> Product_896d7/2
  Product_9d282/1 -> Add_43ae3/2
  Constant_1449.96584011837_c1ff0/1 -> Product_9d282/1
  State_vd_bus_12_691f6/1 -> Product_9d282/2
  Add_25c3a/1 -> Add_43ae3/1
  Constant_1449.96584011837_14eb9/1 -> Product_461d6/1
  State_vd_bus_14_de14e/1 -> Product_461d6/2
  Add_43ae3/1 -> Subtract_29005/1
  Product_461d6/1 -> Subtract_29005/2
  Subtract_29005/1 -> Blockout_d_id_line_12_14_0b4f3/1
